simulink model "SCLAING_TRADITIONAL_21"  (R2021a)
settings: Solver=ode23tb  StartTime=0.0  StopTime=27  MaxStep=1/60  RelTol=1e-2  AbsTol=1e-1  EnableMultiTasking=on
PreLoadFcn:
  | NE39bus_data;
  | PSSMODEL=1;
  | LPSS=0;
  | WAPSS=0;
  | WAPSS2=0;
undefined symbols (not defined in the file): AVR_Data, D1, Delta, line, mac_con, MB, Ns, p0, Pn, s
libraries: spsThreePhaseVIMeasurementLib x40, spsThreePhasePISectionLineLib x34, spsGenericPowerSystemStabilizerLib x20, spsThreePhaseTransformerTwoWindingsLib x12, spsSynchronousMachinepuStandardLib x10, spsExcitationSystemLib x10, spsMultiBandPowerSystemStabilizerLib x10, spsSteamTurbineandGovernorLib x10, slpidlib x10, spsLoadFlowBusLib x9, spsThreePhaseDynamicLoadLib x9, spsThreePhaseParallelRLCLoadLib x9
(part 3 of 4)

== system SCLAING_TRADITIONAL_21/G8 ==
  DFG8 : Inport
  Bus Selector : BusSelector  OutputSignals="Mechanical.Rotor speed deviation  dw (pu)"
  Fcn2 : Fcn  Expr=60*(1+u)
  G8 : spsSynchronousMachinepuStandardLib/Synchronous Machine pu Standard  PresetModel=No  MechanicalLoad=Mechanical power Pm  ShowDetailedParameters=on  RotorType=Round  Units=per unit standard parameters  MeasurementBus=off  NominalParameters="[Pn(8,1)*1e9  22000   50 ]"  Reactances1="[mac_con(8,6:8)  mac_con(8,11:13)  mac_con(8,4)]"  Reactances2=[ 1.305, 0.296, 0.252, 0.474, 0.243, 0.18 ]  dAxisTimeConstants=Open-circuit  qAxisTimeConstants=Open-circuit  TimeConstants1=[]  TimeConstants2="[mac_con(8,9:10)  mac_con(8,14:15)]"  TimeConstants3=[]  TimeConstants4=[]  TimeConstants5=[ 1.01, 0.053, 0.1 ]  TimeConstants6=[]  TimeConstants7=[]  TimeConstants8=[]  StatorResistance=mac_con(8,5)  Mechanical="[ mac_con(8,16)  0  4]"  PolePairs=4  InitialConditions=[0 -25.6939 0.5409 0.5409 0.5409 6.7214 -113.279 126.721 1.90805]  SetSaturation=off  Saturation=[0.6404,0.7127,0.8441,0.9214,0.9956,1.082,1.19,1.316,1.457;0.7,0.7698,0.8872,0.9466,0.9969,1.046,1.1,1.151,1.201]  LoadFlowParameters=[1 540000000 0 0 0]  TsPowergui=0  TsBlock=-1  IterativeModel=Forward Euler  IterativeDiscreteModel=Trapezoidal non iterative  BusType=PV  Pref=p0(8,1)*1E9  Qref=0  Qmin=-inf  Qmax=inf  PLF=0  QLF=0
      settings: SourceProductBaseCode=PS
  M8: Turbine & Regulators : Subsystem
  Matrix Multiply1 : Product  Multiplication=Matrix(*)
  Matrix Multiply2 : Product  Multiplication=Matrix(*)
  PID Controller : slpidlib/PID Controller  Controller=PID  Form=Parallel  TimeDomain=Continuous-time  UseExternalTs=off  SampleTime=-1  IntegratorMethod=Forward Euler  FilterMethod=Forward Euler  ControllerParametersSource=internal  P=-0.20298  I=1  D=0  UseFilter=on  N=100  TunerSelectOption=Frequency Response Based  InitialConditionSource=internal  InitialConditionForIntegrator=0  InitialConditionForFilter=0  DifferentiatorICPrevScaledInput=0  ExternalReset=none  TrackingMode=off  Kt=1  LimitOutput=off  SatLimitsSource=internal  UpperSaturationLimit=inf  LowerSaturationLimit=-inf  LinearizeAsGain=on  AntiWindupMode=none  Kb=1  POutMin=[]  POutMax=[]  IOutMin=[]  IOutMax=[]  DOutMin=[]  DOutMax=[]  NOutMin=[]  NOutMax=[]  SumOutMin=[]  SumOutMax=[]  SaturationOutMin=[]  SaturationOutMax=[]  PParamMin=[]  PParamMax=[]  IParamMin=[]  IParamMax=[]  DParamMin=[]  DParamMax=[]  NParamMin=[]  NParamMax=[]  KbParamMin=[]  KbParamMax=[]  KtParamMin=[]  KtParamMax=[]  KbOutMin=[]  KbOutMax=[]  KtOutMin=[]  KtOutMax=[]  IntegratorOutMin=[]  IntegratorOutMax=[]  FilterOutMin=[]  FilterOutMax=[]  SumI1OutMin=[]  SumI1OutMax=[]  SumI2OutMin=[]  SumI2OutMax=[]  SumI3OutMin=[]  SumI3OutMax=[]  SumI4OutMin=[]  SumI4OutMax=[]  SumDOutMin=[]  SumDOutMax=[]  DifferentiatorOutMin=[]  DifferentiatorOutMax=[]  FilterDiffOutCoefMin=[]  FilterDiffOutCoefMax=[]  ReciprocalOutMin=[]  ReciprocalOutMax=[]  SumDenOutMin=[]  SumDenOutMax=[]  SumNumOutMin=[]  SumNumOutMax=[]  DivideOutMin=[]  DivideOutMax=[]  UdiffTsProdOutMin=[]  UdiffTsProdOutMax=[]  NTsProdOutMin=[]  NTsProdOutMax=[]  UintegralTsProdOutMin=[]  UintegralTsProdOutMax=[]  UngainTsProdOutMin=[]  UngainTsProdOutMax=[]  IntegratorContinuousStateAttributes=''  IntegratorStateMustResolveToSignalObject=off  IntegratorRTWStateStorageClass=Auto  FilterContinuousStateAttributes=''  FilterStateMustResolveToSignalObject=off  FilterRTWStateStorageClass=Auto  ParallelPVariant=InternalParameters  IdealPVariant=Disabled  IVariant=InternalParameters  DVariant=InternalParameters  IntegratorVariant=Continuous  SatVariant=Disabled  AWVariant=Passthrough  PCopyVariant=Disabled  TRVariant=Disabled  FdbkBlocksVariant=Forward  IdealPFdbkVariant=Disabled  SatFdbkVariant=Disabled  DerivativeFilterVariant=ContFilter  NVariant=InternalParameters  NCopyVariant=Disabled  FilterICVariant=InternalICsFilter  IntegratorICVariant=InternalICs  ExternalResetVariant=Disabled  TRSumVariant=Passthrough  SumFdbkVariant=Disabled  SumVariant=Sum_PID  TsampFilterVariant=InternalTs  TsampNgainVariant=Passthrough  TsampIntegralVariant=Passthrough  ExternalSaturationOutDataTypeStr=Inherit: Same as second input
  Pref8 : Constant  Value=0.54
  Scope : Scope
  Sum : Sum  Inputs=|++
  Vref8 : Constant
  A : PMIOPort  Side=Left
  B : PMIOPort  Port=2  Side=Left
  C : PMIOPort  Port=3  Side=Left
  GEN8 : Outport
  wires:
  G8/1 -> M8: Turbine & Regulators/1(m8), Bus Selector/1
  Vref8/1 -> M8: Turbine & Regulators/3(Vref8)
  [PSSmodel] -> M8: Turbine & Regulators/4(PSS8)
  Bus Selector/1 -> PID Controller/1, Fcn2/1  "<Rotor speed deviation  dw (pu)>"
  Fcn2/1 -> GEN8/1, Scope/1
  Pref8/1 -> Sum/1
  Sum/1 -> M8: Turbine & Regulators/2(Pref8)
  PID Controller/1 -> Sum/2
  DFG8/1 -> Matrix Multiply1/1, Matrix Multiply2/1
  M8: Turbine & Regulators/2(Vf8) -> Matrix Multiply2/2
  Matrix Multiply2/1 -> G8/2
  M8: Turbine & Regulators/1(Pm8) -> Matrix Multiply1/2
  Matrix Multiply1/1 -> G8/1
  connections:
  A/RConn1 -- G8/RConn1
  B/RConn1 -- G8/RConn2
  C/RConn1 -- G8/RConn3

== system SCLAING_TRADITIONAL_21/G9 ==
  DFG9 : Inport
  Bus Selector : BusSelector  OutputSignals="Mechanical.Rotor speed deviation  dw (pu)"
  Fcn2 : Fcn  Expr=60*(1+u)
  G9 : spsSynchronousMachinepuStandardLib/Synchronous Machine pu Standard  PresetModel=No  MechanicalLoad=Mechanical power Pm  ShowDetailedParameters=on  RotorType=Round  Units=per unit standard parameters  MeasurementBus=off  NominalParameters="[Pn(9,1)*1E9  22000   50 ]"  Reactances1="[mac_con(9,6:8)  mac_con(9,11:13)  mac_con(9,4)]"  Reactances2=[ 1.305, 0.296, 0.252, 0.474, 0.243, 0.18 ]  dAxisTimeConstants=Open-circuit  qAxisTimeConstants=Open-circuit  TimeConstants1=[]  TimeConstants2="[mac_con(9,9:10)  mac_con(9,14:15)]"  TimeConstants3=[]  TimeConstants4=[]  TimeConstants5=[ 1.01, 0.053, 0.1 ]  TimeConstants6=[]  TimeConstants7=[]  TimeConstants8=[]  StatorResistance=mac_con(9,5)  Mechanical="[ mac_con(9,16)  0  4]"  PolePairs=4  InitialConditions=[0 -16.7125 0.832308 0.832308 0.832308 12.5378 -107.462 132.538 2.08155]  SetSaturation=off  Saturation=[0.6404,0.7127,0.8441,0.9214,0.9956,1.082,1.19,1.316,1.457;0.7,0.7698,0.8872,0.9466,0.9969,1.046,1.1,1.151,1.201]  LoadFlowParameters=[1 830000000 0 0 0]  TsPowergui=0  TsBlock=-1  IterativeModel=Forward Euler  IterativeDiscreteModel=Trapezoidal non iterative  BusType=PV  Pref=p0(9,1)*1E9  Qref=0  Qmin=-inf  Qmax=inf  PLF=0  QLF=0
      settings: SourceProductBaseCode=PS
  "M9: Turbine & Regulators " : Subsystem
  Matrix Multiply1 : Product  Multiplication=Matrix(*)
  Matrix Multiply2 : Product  Multiplication=Matrix(*)
  PID Controller : slpidlib/PID Controller  Controller=PID  Form=Parallel  TimeDomain=Continuous-time  UseExternalTs=off  SampleTime=-1  IntegratorMethod=Forward Euler  FilterMethod=Forward Euler  ControllerParametersSource=internal  P=-0.20298  I=1  D=0  UseFilter=on  N=100  TunerSelectOption=Frequency Response Based  InitialConditionSource=internal  InitialConditionForIntegrator=0  InitialConditionForFilter=0  DifferentiatorICPrevScaledInput=0  ExternalReset=none  TrackingMode=off  Kt=1  LimitOutput=off  SatLimitsSource=internal  UpperSaturationLimit=inf  LowerSaturationLimit=-inf  LinearizeAsGain=on  AntiWindupMode=none  Kb=1  POutMin=[]  POutMax=[]  IOutMin=[]  IOutMax=[]  DOutMin=[]  DOutMax=[]  NOutMin=[]  NOutMax=[]  SumOutMin=[]  SumOutMax=[]  SaturationOutMin=[]  SaturationOutMax=[]  PParamMin=[]  PParamMax=[]  IParamMin=[]  IParamMax=[]  DParamMin=[]  DParamMax=[]  NParamMin=[]  NParamMax=[]  KbParamMin=[]  KbParamMax=[]  KtParamMin=[]  KtParamMax=[]  KbOutMin=[]  KbOutMax=[]  KtOutMin=[]  KtOutMax=[]  IntegratorOutMin=[]  IntegratorOutMax=[]  FilterOutMin=[]  FilterOutMax=[]  SumI1OutMin=[]  SumI1OutMax=[]  SumI2OutMin=[]  SumI2OutMax=[]  SumI3OutMin=[]  SumI3OutMax=[]  SumI4OutMin=[]  SumI4OutMax=[]  SumDOutMin=[]  SumDOutMax=[]  DifferentiatorOutMin=[]  DifferentiatorOutMax=[]  FilterDiffOutCoefMin=[]  FilterDiffOutCoefMax=[]  ReciprocalOutMin=[]  ReciprocalOutMax=[]  SumDenOutMin=[]  SumDenOutMax=[]  SumNumOutMin=[]  SumNumOutMax=[]  DivideOutMin=[]  DivideOutMax=[]  UdiffTsProdOutMin=[]  UdiffTsProdOutMax=[]  NTsProdOutMin=[]  NTsProdOutMax=[]  UintegralTsProdOutMin=[]  UintegralTsProdOutMax=[]  UngainTsProdOutMin=[]  UngainTsProdOutMax=[]  IntegratorContinuousStateAttributes=''  IntegratorStateMustResolveToSignalObject=off  IntegratorRTWStateStorageClass=Auto  FilterContinuousStateAttributes=''  FilterStateMustResolveToSignalObject=off  FilterRTWStateStorageClass=Auto  ParallelPVariant=InternalParameters  IdealPVariant=Disabled  IVariant=InternalParameters  DVariant=InternalParameters  IntegratorVariant=Continuous  SatVariant=Disabled  AWVariant=Passthrough  PCopyVariant=Disabled  TRVariant=Disabled  FdbkBlocksVariant=Forward  IdealPFdbkVariant=Disabled  SatFdbkVariant=Disabled  DerivativeFilterVariant=ContFilter  NVariant=InternalParameters  NCopyVariant=Disabled  FilterICVariant=InternalICsFilter  IntegratorICVariant=InternalICs  ExternalResetVariant=Disabled  TRSumVariant=Passthrough  SumFdbkVariant=Disabled  SumVariant=Sum_PID  TsampFilterVariant=InternalTs  TsampNgainVariant=Passthrough  TsampIntegralVariant=Passthrough  ExternalSaturationOutDataTypeStr=Inherit: Same as second input
  Pref9 : Constant  Value=0.83
  Scope : Scope
  Sum : Sum  Inputs=|++
  Vref9 : Constant
  A : PMIOPort  Side=Left
  B : PMIOPort  Port=2  Side=Left
  C : PMIOPort  Port=3  Side=Left
  Out1 : Outport
  GEN9 : Outport  Port=2
  wires:
  G9/1 -> Bus Selector/1, "M9: Turbine & Regulators "/1(m9)
  [PSSmodel] -> "M9: Turbine & Regulators "/4(PSS9)
  Vref9/1 -> "M9: Turbine & Regulators "/3(Vref9)
  Bus Selector/1 -> PID Controller/1, Fcn2/1  "<Rotor speed deviation  dw (pu)>"
  Fcn2/1 -> GEN9/1, Out1/1, Scope/1
  Pref9/1 -> Sum/1
  Sum/1 -> "M9: Turbine & Regulators "/2(Pref9)
  PID Controller/1 -> Sum/2
  DFG9/1 -> Matrix Multiply2/1, Matrix Multiply1/1
  "M9: Turbine & Regulators "/1(Pm9) -> Matrix Multiply1/2
  Matrix Multiply1/1 -> G9/1
  "M9: Turbine & Regulators "/2(Vf9) -> Matrix Multiply2/2
  Matrix Multiply2/1 -> G9/2
  connections:
  A/RConn1 -- G9/RConn1
  B/RConn1 -- G9/RConn2
  C/RConn1 -- G9/RConn3

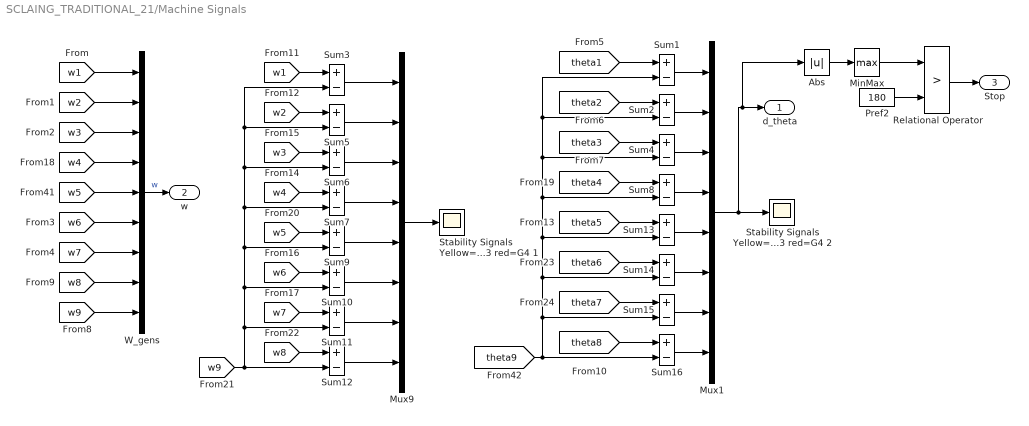
== system SCLAING_TRADITIONAL_21/Machine Signals ==
  Abs : Abs  SaturateOnIntegerOverflow=on
  MinMax : MinMax  Function=max  InputSameDT=on  SaturateOnIntegerOverflow=on
  Mux1 : Mux  Inputs=8
  Mux9 : Mux  Inputs=8
  Pref2 : Constant  Value=180
  Relational Operator : RelationalOperator  Operator=>  RndMeth=Nearest  InputSameDT=on
  Stability Signals Yellow=G1 mag=G2 cyan=G3 red=G4 1 : Scope
  Stability Signals Yellow=G1 mag=G2 cyan=G3 red=G4 2 : Scope
  Sum{1..16} (16 alike) : Sum  Inputs=+-  InputSameDT=on  SaturateOnIntegerOverflow=on  OutDataTypeStr=Inherit: Same as first input
  W_gens : Mux  Inputs=9
  d_theta : Outport
  w : Outport  Port=2
  Stop : Outport  Port=3
  wires:
  Abs/1 -> MinMax/1
  Pref2/1 -> Relational Operator/2
  MinMax/1 -> Relational Operator/1
  W_gens/1 -> w/1  "w"
  Relational Operator/1 -> Stop/1
  Mux9/1 -> Stability Signals Yellow=G1 mag=G2 cyan=G3 red=G4 1/1
  [w1] -> W_gens/1
  [w2] -> W_gens/2
  [w4] -> W_gens/4
  [w3] -> W_gens/3
  [w5] -> W_gens/5
  [w9] -> W_gens/9
  [w8] -> W_gens/8
  [w7] -> W_gens/7
  [w6] -> W_gens/6
  [w1] -> Sum3/1
  [w2] -> Sum5/1
  [w4] -> Sum7/1
  [w3] -> Sum6/1
  [w5] -> Sum9/1
  [w9] -> Sum11/2, Sum10/2, Sum9/2, Sum7/2, Sum6/2, Sum5/2, Sum3/2, Sum12/2
  [w8] -> Sum12/1
  [w7] -> Sum11/1
  [w6] -> Sum10/1
  Sum7/1 -> Mux9/4
  Sum6/1 -> Mux9/3
  Sum5/1 -> Mux9/2
  Sum3/1 -> Mux9/1
  Sum10/1 -> Mux9/6
  Sum9/1 -> Mux9/5
  Sum11/1 -> Mux9/7
  Sum12/1 -> Mux9/8
  [theta9] -> Sum15/2, Sum14/2, Sum4/2, Sum1/2, Sum2/2, Sum8/2, Sum13/2, Sum16/2
  [theta8] -> Sum16/1
  [theta1] -> Sum1/1
  [theta2] -> Sum2/1
  [theta3] -> Sum4/1
  [theta4] -> Sum8/1
  [theta5] -> Sum13/1
  [theta6] -> Sum14/1
  [theta7] -> Sum15/1
  Sum2/1 -> Mux1/2
  Sum1/1 -> Mux1/1
  Sum4/1 -> Mux1/3
  Sum8/1 -> Mux1/4
  Sum13/1 -> Mux1/5
  Sum14/1 -> Mux1/6
  Sum15/1 -> Mux1/7
  Sum16/1 -> Mux1/8
  Mux1/1 -> Abs/1, d_theta/1, Stability Signals Yellow=G1 mag=G2 cyan=G3 red=G4 2/1

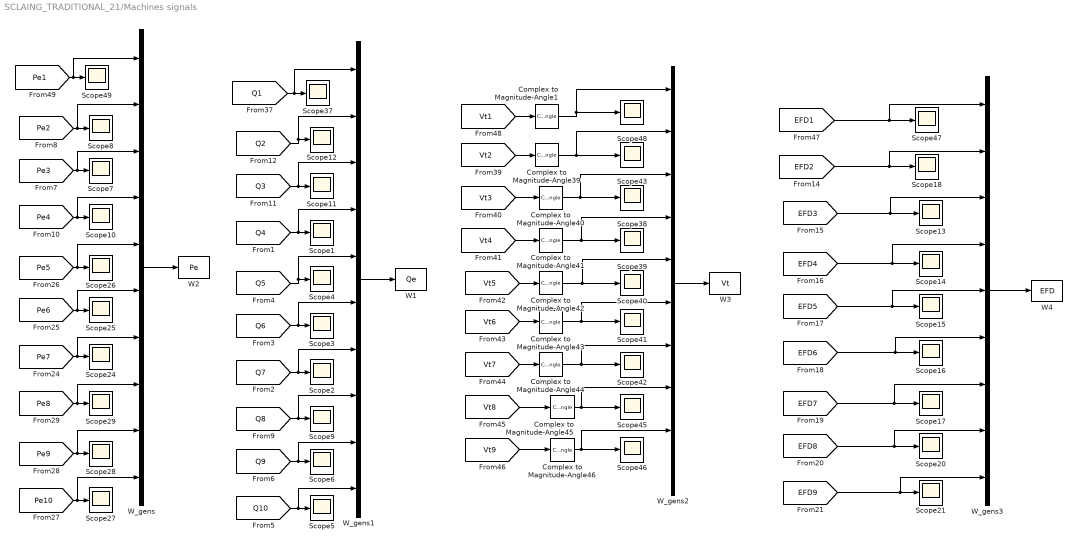
== system SCLAING_TRADITIONAL_21/Machines signals ==
  Complex to Magnitude-Angle{1,39..46} (9 alike) : ComplexToMagnitudeAngle  Output=Magnitude
  Scope{1..18,20..21,24..29,37..43,45..49} (38 alike) : Scope
  W1 : ToWorkspace  VariableName=Qe  SampleTime=1/60
  W2 : ToWorkspace  VariableName=Pe  SampleTime=1/60
  W3 : ToWorkspace  VariableName=Vt  SampleTime=1/60
  W4 : ToWorkspace  VariableName=EFD  SampleTime=1/60
  W_gens : Mux  Inputs=10
  W_gens1 : Mux  Inputs=10
  W_gens2 : Mux  Inputs=10
  W_gens3 : Mux  Inputs=9
  wires:
  [Pe3] -> W_gens/3, Scope7/1
  [Pe2] -> W_gens/2, Scope8/1
  [Vt2] -> Complex to Magnitude-Angle39/1
  Complex to Magnitude-Angle39/1 -> Scope43/1, W_gens2/2
  [Vt3] -> Complex to Magnitude-Angle40/1
  Complex to Magnitude-Angle40/1 -> Scope38/1, W_gens2/3
  [Vt4] -> Complex to Magnitude-Angle41/1
  Complex to Magnitude-Angle41/1 -> Scope39/1, W_gens2/4
  [Vt5] -> Complex to Magnitude-Angle42/1
  Complex to Magnitude-Angle42/1 -> Scope40/1, W_gens2/5
  [Vt6] -> Complex to Magnitude-Angle43/1
  Complex to Magnitude-Angle43/1 -> W_gens2/6, Scope41/1
  [Vt7] -> Complex to Magnitude-Angle44/1
  Complex to Magnitude-Angle44/1 -> Scope42/1, W_gens2/7
  [Vt8] -> Complex to Magnitude-Angle45/1
  Complex to Magnitude-Angle45/1 -> Scope45/1, W_gens2/8
  [Vt9] -> Complex to Magnitude-Angle46/1
  Complex to Magnitude-Angle46/1 -> W_gens2/9, Scope46/1
  [Pe6] -> W_gens/6, Scope25/1
  [Pe5] -> W_gens/5, Scope26/1
  [Pe7] -> W_gens/7, Scope24/1
  [Pe9] -> W_gens/9, Scope28/1
  [Pe8] -> W_gens/8, Scope29/1
  [Pe10] -> W_gens/10, Scope27/1
  [Q3] -> W_gens1/3, Scope11/1
  [Q2] -> W_gens1/2, Scope12/1
  [Q4] -> W_gens1/4, Scope1/1
  [Q6] -> W_gens1/6, Scope3/1
  [Q5] -> W_gens1/5, Scope4/1
  [Q7] -> W_gens1/7, Scope2/1
  [Q9] -> W_gens1/9, Scope6/1
  [Q8] -> W_gens1/8, Scope9/1
  [Q10] -> W_gens1/10, Scope5/1
  [EFD2] -> W_gens3/2, Scope18/1
  [EFD3] -> Scope13/1, W_gens3/3
  [EFD4] -> W_gens3/4, Scope14/1
  [EFD5] -> W_gens3/5, Scope15/1
  [EFD6] -> W_gens3/6, Scope16/1
  [EFD7] -> W_gens3/7, Scope17/1
  [EFD8] -> W_gens3/8, Scope20/1
  [EFD9] -> Scope21/1, W_gens3/9
  [Pe4] -> W_gens/4, Scope10/1
  [Pe1] -> W_gens/1, Scope49/1
  Complex to Magnitude-Angle1/1 -> W_gens2/1, Scope48/1
  [Q1] -> W_gens1/1, Scope37/1
  [EFD1] -> W_gens3/1, Scope47/1
  [Vt1] -> Complex to Magnitude-Angle1/1
  W_gens/1 -> W2/1
  W_gens1/1 -> W1/1
  W_gens2/1 -> W3/1
  W_gens3/1 -> W4/1

== system SCLAING_TRADITIONAL_21/Subsystem1 ==
  In3 : Inport
  Constant16 : Constant  Value=11304000  SampleTime=-1
  Constant17 : Constant  Value=0
  Matrix Multiply5 : Product  Multiplication=Matrix(*)
  Mux1 : Mux  Inputs=2
  Scope34 : Scope
  Sum4 : Sum  Inputs=|++
  Three-Phase Dynamic Load1 : spsThreePhaseDynamicLoadLib/Three-Phase Dynamic Load  NominalVoltage="[ (217684)*1  60 ]"  ActiveReactivePowers=[11304000 0]  PositiveSequence=[0.994 -11.8]  ExternalControl=on  NpNq=[1.3 2]  TimeConstants="[0  0  0  0]"  MinimumVoltage=0.7  Tfilter=-1  LoadFlowParameters=[4,0,0,0,0]
      settings: SourceProductBaseCode=PS
  Uniform Random Number1 : UniformRandomNumber  Minimum=-5e+3  Maximum=5e+3  Seed=1e+4  SampleTime=0.01
  A : PMIOPort  Side=Left
  B : PMIOPort  Port=2  Side=Left
  C : PMIOPort  Port=3  Side=Left
  m : Outport
  wires:
  Constant17/1 -> Mux1/2
  In3/1 -> Matrix Multiply5/1
  Matrix Multiply5/1 -> Scope34/1, Sum4/1
  Uniform Random Number1/1 -> Matrix Multiply5/2
  Three-Phase Dynamic Load1/1 -> m/1
  Sum4/1 -> Mux1/1
  Constant16/1 -> Sum4/2
  Mux1/1 -> Three-Phase Dynamic Load1/1
  connections:
  Three-Phase Dynamic Load1/LConn1 -- A/RConn1
  Three-Phase Dynamic Load1/LConn2 -- B/RConn1
  Three-Phase Dynamic Load1/LConn3 -- C/RConn1

== system SCLAING_TRADITIONAL_21/Subsystem2 ==
  In3 : Inport
  Constant16 : Constant  Value=11304000  SampleTime=-1
  Constant17 : Constant  Value=0
  Matrix Multiply5 : Product  Multiplication=Matrix(*)
  Mux1 : Mux  Inputs=2
  Scope34 : Scope
  Sum4 : Sum  Inputs=|++
  Three-Phase Dynamic Load1 : spsThreePhaseDynamicLoadLib/Three-Phase Dynamic Load  NominalVoltage="[ (217684)*1  60 ]"  ActiveReactivePowers=[11304000 0]  PositiveSequence=[0.994 -11.8]  ExternalControl=on  NpNq=[1.3 2]  TimeConstants="[0  0  0  0]"  MinimumVoltage=0.7  Tfilter=-1  LoadFlowParameters=[4,0,0,0,0]
      settings: SourceProductBaseCode=PS
  Uniform Random Number1 : UniformRandomNumber  Minimum=-5e+3  Maximum=5e+3  Seed=1e+4  SampleTime=0.01
  A : PMIOPort  Side=Left
  B : PMIOPort  Port=2  Side=Left
  C : PMIOPort  Port=3  Side=Left
  m : Outport
  wires:
  Constant17/1 -> Mux1/2
  In3/1 -> Matrix Multiply5/1
  Matrix Multiply5/1 -> Scope34/1, Sum4/1
  Uniform Random Number1/1 -> Matrix Multiply5/2
  Three-Phase Dynamic Load1/1 -> m/1
  Sum4/1 -> Mux1/1
  Constant16/1 -> Sum4/2
  Mux1/1 -> Three-Phase Dynamic Load1/1
  connections:
  Three-Phase Dynamic Load1/LConn1 -- A/RConn1
  Three-Phase Dynamic Load1/LConn2 -- B/RConn1
  Three-Phase Dynamic Load1/LConn3 -- C/RConn1

== system SCLAING_TRADITIONAL_21/Subsystem3 ==
  In3 : Inport
  Constant16 : Constant  Value=11304000  SampleTime=-1
  Constant17 : Constant  Value=0
  Matrix Multiply5 : Product  Multiplication=Matrix(*)
  Mux1 : Mux  Inputs=2
  Scope34 : Scope
  Sum4 : Sum  Inputs=|++
  Three-Phase Dynamic Load1 : spsThreePhaseDynamicLoadLib/Three-Phase Dynamic Load  NominalVoltage="[ (217684)*1  60 ]"  ActiveReactivePowers=[11304000 0]  PositiveSequence=[0.994 -11.8]  ExternalControl=on  NpNq=[1.3 2]  TimeConstants="[0  0  0  0]"  MinimumVoltage=0.7  Tfilter=-1  LoadFlowParameters=[4,0,0,0,0]
      settings: SourceProductBaseCode=PS
  Uniform Random Number1 : UniformRandomNumber  Minimum=-5e+3  Maximum=5e+3  Seed=1e+4  SampleTime=0.01
  A : PMIOPort  Side=Left
  B : PMIOPort  Port=2  Side=Left
  C : PMIOPort  Port=3  Side=Left
  m : Outport
  wires:
  Constant17/1 -> Mux1/2
  In3/1 -> Matrix Multiply5/1
  Matrix Multiply5/1 -> Scope34/1, Sum4/1
  Uniform Random Number1/1 -> Matrix Multiply5/2
  Three-Phase Dynamic Load1/1 -> m/1
  Sum4/1 -> Mux1/1
  Constant16/1 -> Sum4/2
  Mux1/1 -> Three-Phase Dynamic Load1/1
  connections:
  Three-Phase Dynamic Load1/LConn1 -- A/RConn1
  Three-Phase Dynamic Load1/LConn2 -- B/RConn1
  Three-Phase Dynamic Load1/LConn3 -- C/RConn1

== system SCLAING_TRADITIONAL_21/Subsystem4 ==
  In3 : Inport
  Constant16 : Constant  Value=11304000  SampleTime=-1
  Constant17 : Constant  Value=0
  Matrix Multiply5 : Product  Multiplication=Matrix(*)
  Mux1 : Mux  Inputs=2
  Scope34 : Scope
  Sum4 : Sum  Inputs=|++
  Three-Phase Dynamic Load1 : spsThreePhaseDynamicLoadLib/Three-Phase Dynamic Load  NominalVoltage="[ (217684)*1  60 ]"  ActiveReactivePowers=[11304000 0]  PositiveSequence=[0.994 -11.8]  ExternalControl=on  NpNq=[1.3 2]  TimeConstants="[0  0  0  0]"  MinimumVoltage=0.7  Tfilter=-1  LoadFlowParameters=[4,0,0,0,0]
      settings: SourceProductBaseCode=PS
  Uniform Random Number1 : UniformRandomNumber  Minimum=-5e+3  Maximum=5e+3  Seed=1e+4  SampleTime=0.01
  A : PMIOPort  Side=Left
  C : PMIOPort  Port=2  Side=Left
  B : PMIOPort  Port=3  Side=Left
  m : Outport
  wires:
  Constant17/1 -> Mux1/2
  In3/1 -> Matrix Multiply5/1
  Matrix Multiply5/1 -> Scope34/1, Sum4/1
  Uniform Random Number1/1 -> Matrix Multiply5/2
  Three-Phase Dynamic Load1/1 -> m/1
  Sum4/1 -> Mux1/1
  Constant16/1 -> Sum4/2
  Mux1/1 -> Three-Phase Dynamic Load1/1
  connections:
  Three-Phase Dynamic Load1/LConn1 -- A/RConn1
  Three-Phase Dynamic Load1/LConn2 -- B/RConn1
  Three-Phase Dynamic Load1/LConn3 -- C/RConn1

== system SCLAING_TRADITIONAL_21/Subsystem5 ==
  In3 : Inport
  Constant16 : Constant  Value=11304000  SampleTime=-1
  Constant17 : Constant  Value=0
  Matrix Multiply5 : Product  Multiplication=Matrix(*)
  Mux1 : Mux  Inputs=2
  Scope34 : Scope
  Sum4 : Sum  Inputs=|++
  Three-Phase Dynamic Load1 : spsThreePhaseDynamicLoadLib/Three-Phase Dynamic Load  NominalVoltage="[ (217684)*1  60 ]"  ActiveReactivePowers=[11304000 0]  PositiveSequence=[0.994 -11.8]  ExternalControl=on  NpNq=[1.3 2]  TimeConstants="[0  0  0  0]"  MinimumVoltage=0.7  Tfilter=-1  LoadFlowParameters=[4,0,0,0,0]
      settings: SourceProductBaseCode=PS
  Uniform Random Number1 : UniformRandomNumber  Minimum=-5e+3  Maximum=5e+3  Seed=1e+4  SampleTime=0.01
  A : PMIOPort  Side=Left
  B : PMIOPort  Port=2  Side=Left
  C : PMIOPort  Port=3  Side=Left
  m : Outport
  wires:
  Constant17/1 -> Mux1/2
  In3/1 -> Matrix Multiply5/1
  Matrix Multiply5/1 -> Scope34/1, Sum4/1
  Uniform Random Number1/1 -> Matrix Multiply5/2
  Three-Phase Dynamic Load1/1 -> m/1
  Sum4/1 -> Mux1/1
  Constant16/1 -> Sum4/2
  Mux1/1 -> Three-Phase Dynamic Load1/1
  connections:
  Three-Phase Dynamic Load1/LConn1 -- A/RConn1
  Three-Phase Dynamic Load1/LConn2 -- B/RConn1
  Three-Phase Dynamic Load1/LConn3 -- C/RConn1

== system SCLAING_TRADITIONAL_21/Subsystem6 ==
  In3 : Inport
  Constant16 : Constant  Value=11304000  SampleTime=-1
  Constant17 : Constant  Value=0
  Matrix Multiply5 : Product  Multiplication=Matrix(*)
  Mux1 : Mux  Inputs=2
  Scope34 : Scope
  Sum4 : Sum  Inputs=|++
  Three-Phase Dynamic Load1 : spsThreePhaseDynamicLoadLib/Three-Phase Dynamic Load  NominalVoltage="[ (217684)*1  60 ]"  ActiveReactivePowers=[11304000 0]  PositiveSequence=[0.994 -11.8]  ExternalControl=on  NpNq=[1.3 2]  TimeConstants="[0  0  0  0]"  MinimumVoltage=0.7  Tfilter=-1  LoadFlowParameters=[4,0,0,0,0]
      settings: SourceProductBaseCode=PS
  Uniform Random Number1 : UniformRandomNumber  Minimum=-5e+3  Maximum=5e+3  Seed=1e+4  SampleTime=0.01
  A : PMIOPort  Side=Left
  C : PMIOPort  Port=2  Side=Left
  B : PMIOPort  Port=3  Side=Left
  m : Outport
  wires:
  Constant17/1 -> Mux1/2
  In3/1 -> Matrix Multiply5/1
  Matrix Multiply5/1 -> Scope34/1, Sum4/1
  Uniform Random Number1/1 -> Matrix Multiply5/2
  Three-Phase Dynamic Load1/1 -> m/1
  Sum4/1 -> Mux1/1
  Constant16/1 -> Sum4/2
  Mux1/1 -> Three-Phase Dynamic Load1/1
  connections:
  Three-Phase Dynamic Load1/LConn1 -- A/RConn1
  Three-Phase Dynamic Load1/LConn2 -- B/RConn1
  Three-Phase Dynamic Load1/LConn3 -- C/RConn1

== system SCLAING_TRADITIONAL_21/Subsystem7 ==
  In3 : Inport
  Constant16 : Constant  Value=11304000  SampleTime=-1
  Constant17 : Constant  Value=0
  Matrix Multiply5 : Product  Multiplication=Matrix(*)
  Mux1 : Mux  Inputs=2
  Scope34 : Scope
  Sum4 : Sum  Inputs=|++
  Three-Phase Dynamic Load1 : spsThreePhaseDynamicLoadLib/Three-Phase Dynamic Load  NominalVoltage="[ (217684)*1  60 ]"  ActiveReactivePowers=[11304000 0]  PositiveSequence=[0.994 -11.8]  ExternalControl=on  NpNq=[1.3 2]  TimeConstants="[0  0  0  0]"  MinimumVoltage=0.7  Tfilter=-1  LoadFlowParameters=[4,0,0,0,0]
      settings: SourceProductBaseCode=PS
  Uniform Random Number1 : UniformRandomNumber  Minimum=-5e+3  Maximum=5e+3  Seed=1e+4  SampleTime=0.01
  A : PMIOPort  Side=Left
  B : PMIOPort  Port=2  Side=Left
  C : PMIOPort  Port=3  Side=Left
  m : Outport
  wires:
  Constant17/1 -> Mux1/2
  In3/1 -> Matrix Multiply5/1
  Matrix Multiply5/1 -> Scope34/1, Sum4/1
  Uniform Random Number1/1 -> Matrix Multiply5/2
  Three-Phase Dynamic Load1/1 -> m/1
  Sum4/1 -> Mux1/1
  Constant16/1 -> Sum4/2
  Mux1/1 -> Three-Phase Dynamic Load1/1
  connections:
  Three-Phase Dynamic Load1/LConn1 -- A/RConn1
  Three-Phase Dynamic Load1/LConn2 -- B/RConn1
  Three-Phase Dynamic Load1/LConn3 -- C/RConn1

== system SCLAING_TRADITIONAL_21/Subsystem8 ==
  In3 : Inport
  Constant16 : Constant  Value=11304000  SampleTime=-1
  Constant17 : Constant  Value=0
  Matrix Multiply5 : Product  Multiplication=Matrix(*)
  Mux1 : Mux  Inputs=2
  Scope34 : Scope
  Sum4 : Sum  Inputs=|++
  Three-Phase Dynamic Load1 : spsThreePhaseDynamicLoadLib/Three-Phase Dynamic Load  NominalVoltage="[ (217684)*1  60 ]"  ActiveReactivePowers=[11304000 0]  PositiveSequence=[0.994 -11.8]  ExternalControl=on  NpNq=[1.3 2]  TimeConstants="[0  0  0  0]"  MinimumVoltage=0.7  Tfilter=-1  LoadFlowParameters=[4,0,0,0,0]
      settings: SourceProductBaseCode=PS
  Uniform Random Number1 : UniformRandomNumber  Minimum=-5e+3  Maximum=5e+3  Seed=1e+4  SampleTime=0.01
  A : PMIOPort  Side=Left
  B : PMIOPort  Port=2  Side=Left
  C : PMIOPort  Port=3  Side=Left
  m : Outport
  wires:
  Constant17/1 -> Mux1/2
  In3/1 -> Matrix Multiply5/1
  Matrix Multiply5/1 -> Scope34/1, Sum4/1
  Uniform Random Number1/1 -> Matrix Multiply5/2
  Three-Phase Dynamic Load1/1 -> m/1
  Sum4/1 -> Mux1/1
  Constant16/1 -> Sum4/2
  Mux1/1 -> Three-Phase Dynamic Load1/1
  connections:
  Three-Phase Dynamic Load1/LConn1 -- A/RConn1
  Three-Phase Dynamic Load1/LConn2 -- B/RConn1
  Three-Phase Dynamic Load1/LConn3 -- C/RConn1

== system SCLAING_TRADITIONAL_21/Subsystem9 ==
  In3 : Inport
  Constant16 : Constant  Value=11304000  SampleTime=-1
  Constant17 : Constant  Value=0
  Matrix Multiply5 : Product  Multiplication=Matrix(*)
  Mux1 : Mux  Inputs=2
  Scope34 : Scope
  Sum4 : Sum  Inputs=|++
  Three-Phase Dynamic Load1 : spsThreePhaseDynamicLoadLib/Three-Phase Dynamic Load  NominalVoltage="[ (217684)*1  60 ]"  ActiveReactivePowers=[11304000 0]  PositiveSequence=[0.994 -11.8]  ExternalControl=on  NpNq=[1.3 2]  TimeConstants="[0  0  0  0]"  MinimumVoltage=0.7  Tfilter=-1  LoadFlowParameters=[4,0,0,0,0]
      settings: SourceProductBaseCode=PS
  Uniform Random Number1 : UniformRandomNumber  Minimum=-5e+3  Maximum=5e+3  Seed=1e+4  SampleTime=0.01
  A : PMIOPort  Side=Left
  C : PMIOPort  Port=2  Side=Left
  B : PMIOPort  Port=3  Side=Left
  m : Outport
  wires:
  Constant17/1 -> Mux1/2
  In3/1 -> Matrix Multiply5/1
  Matrix Multiply5/1 -> Scope34/1, Sum4/1
  Uniform Random Number1/1 -> Matrix Multiply5/2
  Three-Phase Dynamic Load1/1 -> m/1
  Sum4/1 -> Mux1/1
  Constant16/1 -> Sum4/2
  Mux1/1 -> Three-Phase Dynamic Load1/1
  connections:
  Three-Phase Dynamic Load1/LConn1 -- A/RConn1
  Three-Phase Dynamic Load1/LConn2 -- B/RConn1
  Three-Phase Dynamic Load1/LConn3 -- C/RConn1

== system SCLAING_TRADITIONAL_21/System Data ==
  ->pu : Gain  Gain=1/(230e3/sqrt(3)*sqrt(2))  SaturateOnIntegerOverflow=on  OutDataTypeStr=Inherit: Same as input  ParamDataTypeStr=Inherit: Same as input
  3-Phase Active & Reactive Power (Phasor Type) : powerlib_extras/Phasor Library/3-Phase Active & Reactive Power (Phasor Type)
      settings: SourceProductBaseCode=PS
  Complex to Magnitude-Angle : ComplexToMagnitudeAngle  Output=Magnitude
  Complex to Magnitude-Angle1 : ComplexToMagnitudeAngle  Output=Magnitude
  Mux : Mux  Inputs=2
  P34 : Gain  Gain=1e-6  SaturateOnIntegerOverflow=on  OutDataTypeStr=Inherit: Same as input  ParamDataTypeStr=Inherit: Same as input
  Selector : Selector  InputPortWidth=2  IndexOptions=Index vector (dialog)  Indices=1  OutputSizes=1
  Sequence Analyzer (Phasor Type) : powerlib_extras/Phasor Library/Sequence Analyzer (Phasor Type)  seq=Positive
      settings: SourceProductBaseCode=PS
  Sequence Analyzer (Phasor Type)1 : powerlib_extras/Phasor Library/Sequence Analyzer (Phasor Type)  seq=Positive
      settings: SourceProductBaseCode=PS
  Terminator1 : Terminator
  Terminator2 : Terminator
  Vabc_B3 : Scope
  Vabc_B4 : Scope
  W2 : ToWorkspace  VariableName=P21  SampleTime=1/60
  Vps : Outport
  p34 : Outport  Port=2
  wires:
  [Vabc_B4] -> Sequence Analyzer (Phasor Type)/1, 3-Phase Active & Reactive Power (Phasor Type)/1, Complex to Magnitude-Angle/1
  [Vabc_B3] -> Sequence Analyzer (Phasor Type)1/1, Complex to Magnitude-Angle1/1
  Sequence Analyzer (Phasor Type)/2 -> Terminator1/1
  Sequence Analyzer (Phasor Type)1/2 -> Terminator2/1
  Sequence Analyzer (Phasor Type)1/1 -> Mux/2
  [Iabc_B4] -> 3-Phase Active & Reactive Power (Phasor Type)/2
  3-Phase Active & Reactive Power (Phasor Type)/1 -> Selector/1
  ->pu/1 -> Vps/1
  Sequence Analyzer (Phasor Type)/1 -> Mux/1
  Mux/1 -> ->pu/1
  P34/1 -> p34/1, W2/1
  Complex to Magnitude-Angle/1 -> Vabc_B4/1
  Complex to Magnitude-Angle1/1 -> Vabc_B3/1
  Selector/1 -> P34/1

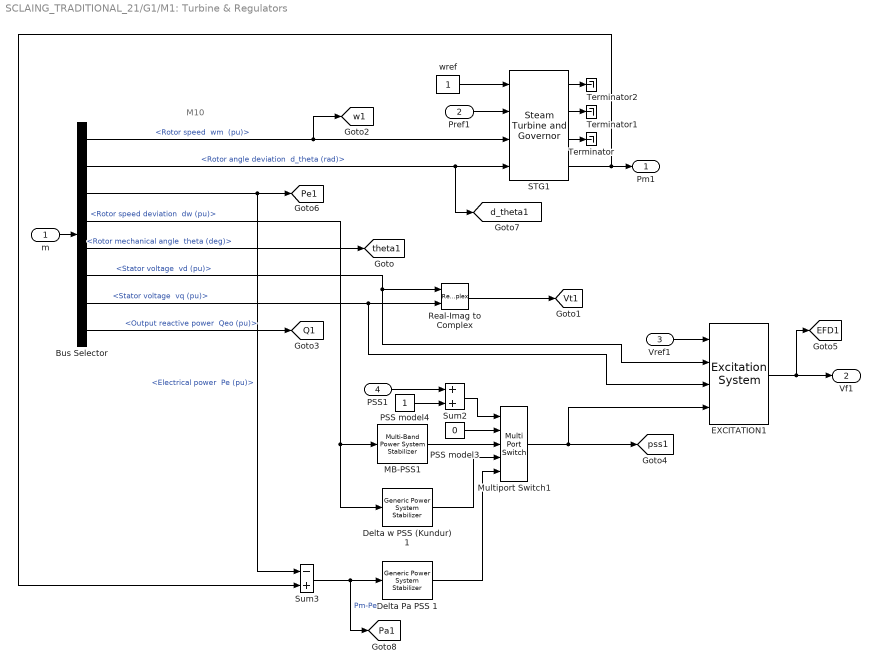
== system SCLAING_TRADITIONAL_21/G1/M1: Turbine & Regulators ==
  note: M10
  m : Inport
  Pref1 : Inport  Port=2
  Vref1 : Inport  Port=3
  PSS1 : Inport  Port=4
  Bus Selector : BusSelector  OutputSignals="Mechanical.Rotor speed  wm  (pu),Mechanical.Rotor angle deviation  d_theta (rad),Mechanical.Electrical power  Pe (pu),Mechanical.Rotor speed deviation  dw (pu),Mechanical.Rotor mechanical angle  theta (deg),dq0 components.Stator voltage  vd (pu),dq0 components.Stator voltage  vq (pu),Output reactive power  Qeo (pu)"
  Delta Pa PSS 1 : spsGenericPowerSystemStabilizerLib/Generic Power System Stabilizer  Tsensor=15e-3  K=2.5*1.25  Twashout=1  Tleadlag1=[60e-3 1]  Tleadlag2=[0 0]  VSlimits=[-0.15 0.15]  Vinit=0  Plot_On=off  MagdB_On=on  FreqRange=logspace(-2,2,500)
      settings: SourceProductBaseCode=PS
  Delta w PSS (Kundur) 1 : spsGenericPowerSystemStabilizerLib/Generic Power System Stabilizer  Tsensor=15e-3  K=30  Twashout=10  Tleadlag1=[50e-3 20e-3]  Tleadlag2=[3 5.4]  VSlimits=[-0.15 0.15]  Vinit=0  Plot_On=off  MagdB_On=on  FreqRange=logspace(-2,2,500)
      settings: SourceProductBaseCode=PS
  EXCITATION1 : spsExcitationSystemLib/Excitation System  tr=AVR_Data(1,1)  reg=[ AVR_Data(1,2:3) ]  exc=[ 1, 0 ]  tgr=[ AVR_Data(1,4:5)]  damp=[ 0, 0 ]  sat=[ 0, 0 ]  lim="[ AVR_Data(1,7:8)  0 ]"  v0=[1,1.07168]
      settings: SourceProductBaseCode=PS
  MB-PSS1 : spsMultiBandPowerSystemStabilizerLib/Multi-Band Power System Stabilizer  OperationMode=Simplified settings  Kg=MB(1)  GL=[MB(2) MB(3)]  GI=[MB(4) MB(5)]  GH=[MB(6) MB(7)]  GLd=[66 66 9.4]  TcLF=[1.667 2 0 0 0 0 2 2.4 0 0 0 0 1 1]  GId=[66 66 47.6]  TcIF=[1 1 0.25 0.3 0 0 1 1 0.3 0.36 0 0 0 0]  GHd=[66 66 233]  TcHF="[0.01 0.012 0 0 0 0  0.012 0.0144 0 0 0 0 1 1]"  LIM=[.075 .15 .15 .15]  Plot_On=off  MagdB_On=off  FreqRange=logspace(-2,2,500)
      settings: SourceProductBaseCode=PS
  Multiport Switch1 : MultiPortSwitch  Inputs=4  InputSameDT=on
  PSS model3 : Constant  Value=0
  PSS model4 : Constant
  Real-Imag to Complex : RealImagToComplex
  STG1 : spsSteamTurbineandGovernorLib/Steam Turbine and Governor  gentype=Tandem-compound (single mass)  reg1="[ 1  0.05    0 ]"  reg2="[ 0.001  0.15 ]"  reg3="[ -0.1  0.1  0  4.496 ]"  N=Ns  turb1="[ 0  10   3.3   0.5   ]"  turb2="[   0   0.36    0.36   0.28   ]"  HA="[ 0.046  1.430  1.465   0.192 ]"  KA="[ 90.44  53.88  64.59   62.94  ]"  DA="[ 0.0115  0.3575  0.3663   0.0137  ]"  ini1=1  ini2=[0.779316,-31.4247]
      settings: SourceProductBaseCode=PS
  Sum2 : Sum  InputSameDT=on  SaturateOnIntegerOverflow=on  OutDataTypeStr=Inherit: Same as first input
  Sum3 : Sum  Inputs=-+  InputSameDT=on  SaturateOnIntegerOverflow=on  OutDataTypeStr=Inherit: Same as first input
  Terminator : Terminator
  Terminator1 : Terminator
  Terminator2 : Terminator
  wref : Constant
  Pm1 : Outport  InitialOutput=0
  Vf1 : Outport  Port=2  InitialOutput=0
  tag scope: EFD1=global, Pa1=global, Pe1=global, Q1=global, Vt1=global, d_theta1=global, pss1=global, theta1=global, w1=global
  wires:
  Bus Selector/7 -> EXCITATION1/3, Real-Imag to Complex/2  "<Stator voltage  vq (pu)>"
  wref/1 -> STG1/1
  Pref1/1 -> STG1/2
  m/1 -> Bus Selector/1
  Vref1/1 -> EXCITATION1/1
  EXCITATION1/1 -> Vf1/1, [EFD1]
  Real-Imag to Complex/1 -> [Vt1]
  Bus Selector/5 -> [theta1]  "<Rotor mechanical angle  theta (deg)>"
  Bus Selector/6 -> Real-Imag to Complex/1, EXCITATION1/2  "<Stator voltage  vd (pu)>"
  STG1/3 -> Terminator/1
  STG1/4 -> Sum3/2, Pm1/1
  STG1/2 -> Terminator1/1
  STG1/1 -> Terminator2/1
  Bus Selector/1 -> [w1], STG1/3  "<Rotor speed  wm  (pu)>"
  Bus Selector/2 -> [d_theta1], STG1/4  "<Rotor angle deviation  d_theta (rad)>"
  Bus Selector/3 -> Sum3/1, [Pe1]  "<Electrical power  Pe (pu)>"
  Bus Selector/8 -> [Q1]  "<Output reactive power  Qeo (pu)>"
  Sum3/1 -> [Pa1], Delta Pa PSS 1/1  "Pm-Pe"
  PSS1/1 -> Sum2/1
  Sum2/1 -> Multiport Switch1/1
  PSS model4/1 -> Sum2/2
  Delta Pa PSS 1/1 -> Multiport Switch1/5
  Delta w PSS (Kundur) 1/1 -> Multiport Switch1/4
  MB-PSS1/1 -> Multiport Switch1/3
  PSS model3/1 -> Multiport Switch1/2
  Multiport Switch1/1 -> [pss1], EXCITATION1/4
  Bus Selector/4 -> Delta w PSS (Kundur) 1/1, MB-PSS1/1  "<Rotor speed deviation  dw (pu)>"

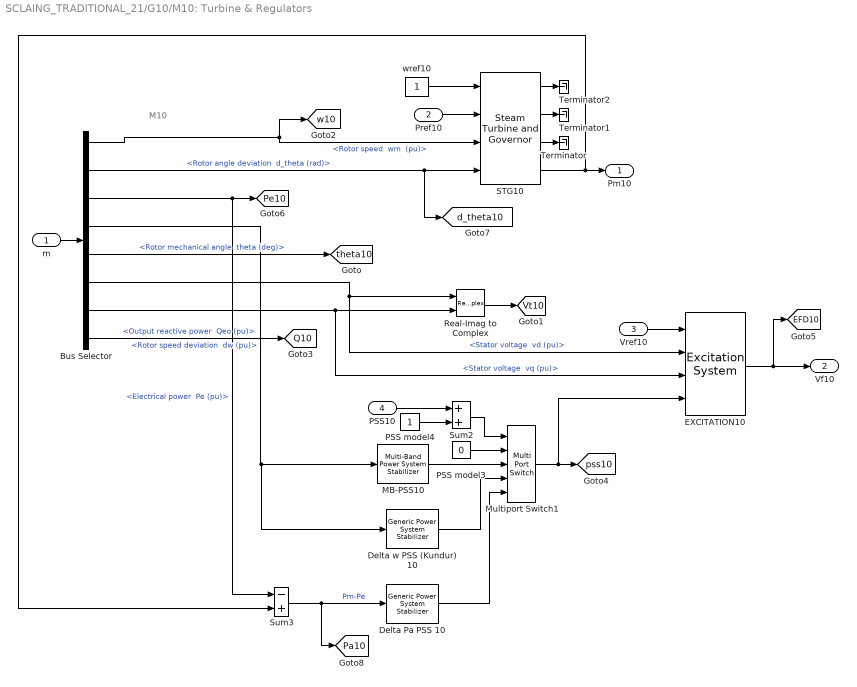
== system SCLAING_TRADITIONAL_21/G10/M10: Turbine & Regulators ==
  note: M10
  m : Inport
  Pref10 : Inport  Port=2
  Vref10 : Inport  Port=3
  PSS10 : Inport  Port=4
  Bus Selector : BusSelector  OutputSignals="Mechanical.Rotor speed  wm  (pu),Mechanical.Rotor angle deviation  d_theta (rad),Mechanical.Electrical power  Pe (pu),Mechanical.Rotor speed deviation  dw (pu),Mechanical.Rotor mechanical angle  theta (deg),dq0 components.Stator voltage  vd (pu),dq0 components.Stator voltage  vq (pu),Output reactive power  Qeo (pu)"
  Delta Pa PSS 10 : spsGenericPowerSystemStabilizerLib/Generic Power System Stabilizer  Tsensor=15e-3  K=2.5*1.25  Twashout=1  Tleadlag1=[60e-3 1]  Tleadlag2=[0 0]  VSlimits=[-0.15 0.15]  Vinit=0  Plot_On=off  MagdB_On=on  FreqRange=logspace(-2,2,500)
      settings: SourceProductBaseCode=PS
  Delta w PSS (Kundur) 10 : spsGenericPowerSystemStabilizerLib/Generic Power System Stabilizer  Tsensor=15e-3  K=30  Twashout=10  Tleadlag1=[50e-3 20e-3]  Tleadlag2=[3 5.4]  VSlimits=[-0.15 0.15]  Vinit=0  Plot_On=off  MagdB_On=on  FreqRange=logspace(-2,2,500)
      settings: SourceProductBaseCode=PS
  EXCITATION10 : spsExcitationSystemLib/Excitation System  tr=AVR_Data(1,1)  reg=[ AVR_Data(1,2:3) ]  exc=[ 1, 0 ]  tgr=[ AVR_Data(1,4:5)]  damp=[ 0, 0 ]  sat=[ 0, 0 ]  lim="[ AVR_Data(1,7:8)  0 ]"  v0=[1,1.1157]
      settings: SourceProductBaseCode=PS
  "MB-PSS10 " : spsMultiBandPowerSystemStabilizerLib/Multi-Band Power System Stabilizer  OperationMode=Simplified settings  Kg=MB(1)  GL=[MB(2) MB(3)]  GI=[MB(4) MB(5)]  GH=[MB(6) MB(7)]  GLd=[66 66 9.4]  TcLF=[1.667 2 0 0 0 0 2 2.4 0 0 0 0 1 1]  GId=[66 66 47.6]  TcIF=[1 1 0.25 0.3 0 0 1 1 0.3 0.36 0 0 0 0]  GHd=[66 66 233]  TcHF="[0.01 0.012 0 0 0 0  0.012 0.0144 0 0 0 0 1 1]"  LIM=[.075 .15 .15 .15]  Plot_On=off  MagdB_On=off  FreqRange=logspace(-2,2,500)
      settings: SourceProductBaseCode=PS
  Multiport Switch1 : MultiPortSwitch  Inputs=4  InputSameDT=on
  PSS model3 : Constant  Value=0
  PSS model4 : Constant
  Real-Imag to Complex : RealImagToComplex
  STG10 : spsSteamTurbineandGovernorLib/Steam Turbine and Governor  gentype=Tandem-compound (single mass)  reg1="[ 1  0.05    0 ]"  reg2="[ 0.001  0.15 ]"  reg3="[ -0.1  0.1  0  4.496 ]"  N=Ns  turb1="[ 0  10   3.3   0.5   ]"  turb2="[   0   0.36    0.36   0.28   ]"  HA="[ 0.046  1.430  1.465   0.192 ]"  KA="[ 90.44  53.88  64.59   62.94  ]"  DA="[ 0.0115  0.3575  0.3663   0.0137  ]"  ini1=0.25  ini2=[0.779316,-31.4247]
      settings: SourceProductBaseCode=PS
  Sum2 : Sum  InputSameDT=on  SaturateOnIntegerOverflow=on  OutDataTypeStr=Inherit: Same as first input
  Sum3 : Sum  Inputs=-+  InputSameDT=on  SaturateOnIntegerOverflow=on  OutDataTypeStr=Inherit: Same as first input
  Terminator : Terminator
  Terminator1 : Terminator
  Terminator2 : Terminator
  wref10 : Constant
  Pm10 : Outport  InitialOutput=0
  Vf10 : Outport  Port=2  InitialOutput=0
  tag scope: EFD10=global, Pa10=global, Pe10=global, Q10=global, Vt10=global, d_theta10=global, pss10=global, theta10=global, w10=global
  wires:
  Bus Selector/7 -> EXCITATION10/3, Real-Imag to Complex/2  "<Stator voltage  vq (pu)>"
  wref10/1 -> STG10/1
  Pref10/1 -> STG10/2
  m/1 -> Bus Selector/1
  Vref10/1 -> EXCITATION10/1
  EXCITATION10/1 -> Vf10/1, [EFD10]
  Real-Imag to Complex/1 -> [Vt10]
  Bus Selector/5 -> [theta10]  "<Rotor mechanical angle  theta (deg)>"
  Bus Selector/6 -> Real-Imag to Complex/1, EXCITATION10/2  "<Stator voltage  vd (pu)>"
  STG10/3 -> Terminator/1
  STG10/4 -> Sum3/2, Pm10/1
  STG10/2 -> Terminator1/1
  STG10/1 -> Terminator2/1
  Bus Selector/1 -> STG10/3, [w10]  "<Rotor speed  wm  (pu)>"
  Bus Selector/2 -> [d_theta10], STG10/4  "<Rotor angle deviation  d_theta (rad)>"
  Bus Selector/3 -> Sum3/1, [Pe10]  "<Electrical power  Pe (pu)>"
  Bus Selector/4 -> Delta w PSS (Kundur) 10/1, "MB-PSS10 "/1  "<Rotor speed deviation  dw (pu)>"
  Bus Selector/8 -> [Q10]  "<Output reactive power  Qeo (pu)>"
  Sum3/1 -> Delta Pa PSS 10/1, [Pa10]  "Pm-Pe"
  Sum2/1 -> Multiport Switch1/1
  PSS model4/1 -> Sum2/2
  Delta Pa PSS 10/1 -> Multiport Switch1/5
  Delta w PSS (Kundur) 10/1 -> Multiport Switch1/4
  "MB-PSS10 "/1 -> Multiport Switch1/3
  PSS model3/1 -> Multiport Switch1/2
  Multiport Switch1/1 -> EXCITATION10/4, [pss10]
  PSS10/1 -> Sum2/1

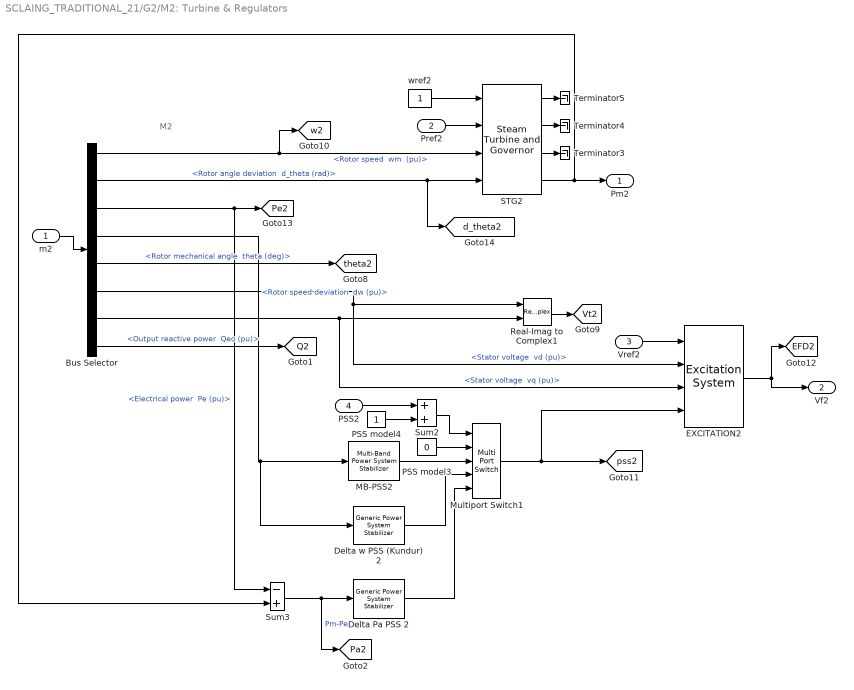
== system SCLAING_TRADITIONAL_21/G2/M2: Turbine & Regulators ==
  note: M2
  m2 : Inport
  Pref2 : Inport  Port=2
  Vref2 : Inport  Port=3
  PSS2 : Inport  Port=4
  Bus Selector : BusSelector  OutputSignals="Mechanical.Rotor speed  wm  (pu),Mechanical.Rotor angle deviation  d_theta (rad),Mechanical.Electrical power  Pe (pu),Mechanical.Rotor speed deviation  dw (pu),Mechanical.Rotor mechanical angle  theta (deg),dq0 components.Stator voltage  vd (pu),dq0 components.Stator voltage  vq (pu),Output reactive power  Qeo (pu)"
  Delta Pa PSS 2 : spsGenericPowerSystemStabilizerLib/Generic Power System Stabilizer  Tsensor=15e-3  K=2.5*1.25  Twashout=1  Tleadlag1=[60e-3 1]  Tleadlag2=[0 0]  VSlimits=[-0.15 0.15]  Vinit=0  Plot_On=off  MagdB_On=on  FreqRange=logspace(-2,2,500)
      settings: SourceProductBaseCode=PS
  Delta w PSS (Kundur) 2 : spsGenericPowerSystemStabilizerLib/Generic Power System Stabilizer  Tsensor=15e-3  K=30  Twashout=10  Tleadlag1=[50e-3 20e-3]  Tleadlag2=[3 5.4]  VSlimits=[-0.15 0.15]  Vinit=0  Plot_On=off  MagdB_On=on  FreqRange=logspace(-2,2,500)
      settings: SourceProductBaseCode=PS
  EXCITATION2 : spsExcitationSystemLib/Excitation System  tr=AVR_Data(2,1)  reg=[ AVR_Data(2,2:3) ]  exc=[ 1, 0 ]  tgr=[ AVR_Data(2,4:5)]  damp=[ 0, 0 ]  sat=[ 0, 0 ]  lim="[ AVR_Data(2,7:8)  0 ]"  v0=[1,1.77729]
      settings: SourceProductBaseCode=PS
  MB-PSS2 : spsMultiBandPowerSystemStabilizerLib/Multi-Band Power System Stabilizer  OperationMode=Simplified settings  Kg=MB(1)  GL=[MB(2) MB(3)]  GI=[MB(4) MB(5)]  GH=[MB(6) MB(7)]  GLd=[66 66 9.4]  TcLF=[1.667 2 0 0 0 0 2 2.4 0 0 0 0 1 1]  GId=[66 66 47.6]  TcIF=[1 1 0.25 0.3 0 0 1 1 0.3 0.36 0 0 0 0]  GHd=[66 66 233]  TcHF="[0.01 0.012 0 0 0 0  0.012 0.0144 0 0 0 0 1 1]"  LIM=[.075 .15 .15 .15]  Plot_On=off  MagdB_On=off  FreqRange=logspace(-2,2,500)
      settings: SourceProductBaseCode=PS
  Multiport Switch1 : MultiPortSwitch  Inputs=4  InputSameDT=on
  PSS model3 : Constant  Value=0
  PSS model4 : Constant
  Real-Imag to Complex1 : RealImagToComplex
  STG2 : spsSteamTurbineandGovernorLib/Steam Turbine and Governor  gentype=Tandem-compound (single mass)  reg1="[ 1  0.05    0 ]"  reg2="[ 0.001  0.15 ]"  reg3="[ -0.1  0.1  0  4.496 ]"  N=Ns  turb1="[ 0  10   3.3   0.5   ]"  turb2="[   0   0.36    0.36   0.28   ]"  HA="[ 0.046  1.430  1.465   0.192 ]"  KA="[ 90.44  53.88  64.59   62.94  ]"  DA="[ 0.0115  0.3575  0.3663   0.0137  ]"  ini1=0.277303  ini2=[0.779316,-31.4247]
      settings: SourceProductBaseCode=PS
  Sum2 : Sum  InputSameDT=on  SaturateOnIntegerOverflow=on  OutDataTypeStr=Inherit: Same as first input
  Sum3 : Sum  Inputs=-+  InputSameDT=on  SaturateOnIntegerOverflow=on  OutDataTypeStr=Inherit: Same as first input
  Terminator3 : Terminator
  Terminator4 : Terminator
  Terminator5 : Terminator
  wref2 : Constant
  Pm2 : Outport  InitialOutput=0
  Vf2 : Outport  Port=2  InitialOutput=0
  tag scope: EFD2=global, Pa2=global, Pe2=global, Q2=global, Vt2=global, d_theta2=global, pss2=global, theta2=global, w2=global
  wires:
  Bus Selector/7 -> EXCITATION2/3, Real-Imag to Complex1/2  "<Stator voltage  vq (pu)>"
  wref2/1 -> STG2/1
  Pref2/1 -> STG2/2
  m2/1 -> Bus Selector/1
  Vref2/1 -> EXCITATION2/1
  EXCITATION2/1 -> Vf2/1, [EFD2]
  Real-Imag to Complex1/1 -> [Vt2]
  Bus Selector/5 -> [theta2]  "<Rotor mechanical angle  theta (deg)>"
  Bus Selector/6 -> EXCITATION2/2, Real-Imag to Complex1/1  "<Stator voltage  vd (pu)>"
  STG2/3 -> Terminator3/1
  STG2/4 -> Sum3/2, Pm2/1
  STG2/2 -> Terminator4/1
  STG2/1 -> Terminator5/1
  Bus Selector/1 -> [w2], STG2/3  "<Rotor speed  wm  (pu)>"
  Bus Selector/2 -> [d_theta2], STG2/4  "<Rotor angle deviation  d_theta (rad)>"
  Bus Selector/3 -> Sum3/1, [Pe2]  "<Electrical power  Pe (pu)>"
  Bus Selector/4 -> Delta w PSS (Kundur) 2/1, MB-PSS2/1  "<Rotor speed deviation  dw (pu)>"
  Bus Selector/8 -> [Q2]  "<Output reactive power  Qeo (pu)>"
  Sum3/1 -> [Pa2], Delta Pa PSS 2/1  "Pm-Pe"
  Sum2/1 -> Multiport Switch1/1
  PSS model4/1 -> Sum2/2
  Delta Pa PSS 2/1 -> Multiport Switch1/5
  Delta w PSS (Kundur) 2/1 -> Multiport Switch1/4
  MB-PSS2/1 -> Multiport Switch1/3
  PSS model3/1 -> Multiport Switch1/2
  Multiport Switch1/1 -> [pss2], EXCITATION2/4
  PSS2/1 -> Sum2/1

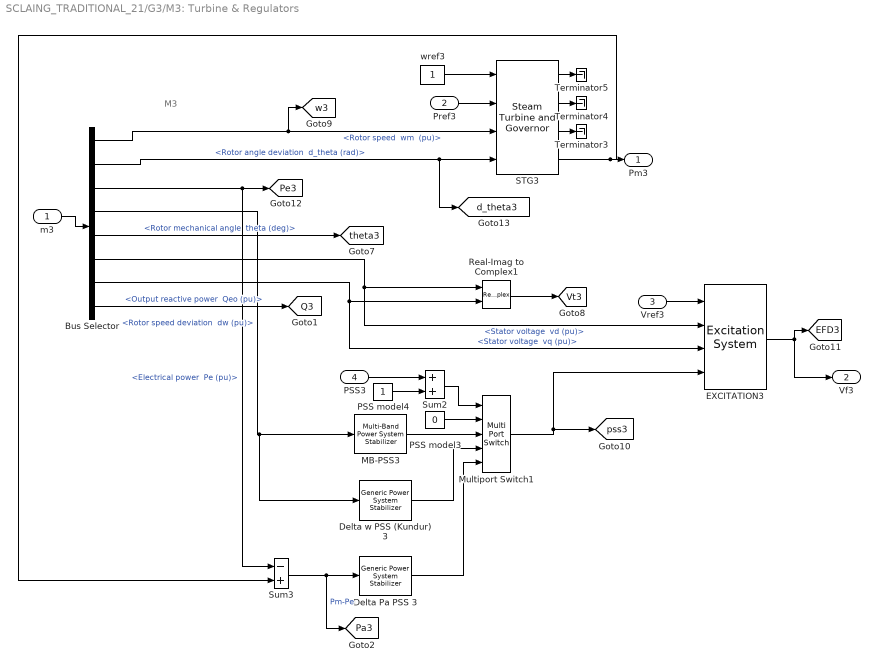
== system SCLAING_TRADITIONAL_21/G3/M3: Turbine & Regulators ==
  note: M3
  m3 : Inport
  Pref3 : Inport  Port=2
  Vref3 : Inport  Port=3
  PSS3 : Inport  Port=4
  Bus Selector : BusSelector  OutputSignals="Mechanical.Rotor speed  wm  (pu),Mechanical.Rotor angle deviation  d_theta (rad),Mechanical.Electrical power  Pe (pu),Mechanical.Rotor speed deviation  dw (pu),Mechanical.Rotor mechanical angle  theta (deg),dq0 components.Stator voltage  vd (pu),dq0 components.Stator voltage  vq (pu),Output reactive power  Qeo (pu)"
  Delta Pa PSS 3 : spsGenericPowerSystemStabilizerLib/Generic Power System Stabilizer  Tsensor=15e-3  K=2.5*1.25  Twashout=1  Tleadlag1=[60e-3 1]  Tleadlag2=[0 0]  VSlimits=[-0.15 0.15]  Vinit=0  Plot_On=off  MagdB_On=on  FreqRange=logspace(-2,2,500)
      settings: SourceProductBaseCode=PS
  Delta w PSS (Kundur) 3 : spsGenericPowerSystemStabilizerLib/Generic Power System Stabilizer  Tsensor=15e-3  K=30  Twashout=10  Tleadlag1=[50e-3 20e-3]  Tleadlag2=[3 5.4]  VSlimits=[-0.15 0.15]  Vinit=0  Plot_On=off  MagdB_On=on  FreqRange=logspace(-2,2,500)
      settings: SourceProductBaseCode=PS
  EXCITATION3 : spsExcitationSystemLib/Excitation System  tr=AVR_Data(3,1)  reg=[ AVR_Data(3,2:3) ]  exc=[ 1, 0 ]  tgr=[ AVR_Data(3,4:5)]  damp=[ 0, 0 ]  sat=[ 0, 0 ]  lim="[ AVR_Data(3,7:8)  0 ]"  v0=[1,2.25944]
      settings: SourceProductBaseCode=PS
  MB-PSS3 : spsMultiBandPowerSystemStabilizerLib/Multi-Band Power System Stabilizer  OperationMode=Simplified settings  Kg=MB(1)  GL=[MB(2) MB(3)]  GI=[MB(4) MB(5)]  GH=[MB(6) MB(7)]  GLd=[66 66 9.4]  TcLF=[1.667 2 0 0 0 0 2 2.4 0 0 0 0 1 1]  GId=[66 66 47.6]  TcIF=[1 1 0.25 0.3 0 0 1 1 0.3 0.36 0 0 0 0]  GHd=[66 66 233]  TcHF="[0.01 0.012 0 0 0 0  0.012 0.0144 0 0 0 0 1 1]"  LIM=[.075 .15 .15 .15]  Plot_On=off  MagdB_On=off  FreqRange=logspace(-2,2,500)
      settings: SourceProductBaseCode=PS
  Multiport Switch1 : MultiPortSwitch  Inputs=4  InputSameDT=on
  PSS model3 : Constant  Value=0
  PSS model4 : Constant
  Real-Imag to Complex1 : RealImagToComplex
  STG3 : spsSteamTurbineandGovernorLib/Steam Turbine and Governor  gentype=Tandem-compound (single mass)  reg1="[ 1  0.05    0 ]"  reg2="[ 0.001  0.15 ]"  reg3="[ -0.1  0.1  0  4.496 ]"  N=Ns  turb1="[ 0  10   3.3   0.5   ]"  turb2="[   0   0.36    0.36   0.28   ]"  HA="[ 0.046  1.430  1.465   0.192 ]"  KA="[ 90.44  53.88  64.59   62.94  ]"  DA="[ 0.0115  0.3575  0.3663   0.0137  ]"  ini1=0.65  ini2=[0.779316,-31.4247]
      settings: SourceProductBaseCode=PS
  Sum2 : Sum  InputSameDT=on  SaturateOnIntegerOverflow=on  OutDataTypeStr=Inherit: Same as first input
  Sum3 : Sum  Inputs=-+  InputSameDT=on  SaturateOnIntegerOverflow=on  OutDataTypeStr=Inherit: Same as first input
  Terminator3 : Terminator
  Terminator4 : Terminator
  Terminator5 : Terminator
  wref3 : Constant
  Pm3 : Outport  InitialOutput=0
  Vf3 : Outport  Port=2  InitialOutput=0
  tag scope: EFD3=global, Pa3=global, Pe3=global, Q3=global, Vt3=global, d_theta3=global, pss3=global, theta3=global, w3=global
  wires:
  Bus Selector/7 -> EXCITATION3/3, Real-Imag to Complex1/2  "<Stator voltage  vq (pu)>"
  wref3/1 -> STG3/1
  Pref3/1 -> STG3/2
  m3/1 -> Bus Selector/1
  Vref3/1 -> EXCITATION3/1
  EXCITATION3/1 -> Vf3/1, [EFD3]
  Real-Imag to Complex1/1 -> [Vt3]
  Bus Selector/5 -> [theta3]  "<Rotor mechanical angle  theta (deg)>"
  Bus Selector/6 -> EXCITATION3/2, Real-Imag to Complex1/1  "<Stator voltage  vd (pu)>"
  STG3/3 -> Terminator3/1
  STG3/4 -> Sum3/2, Pm3/1
  STG3/2 -> Terminator4/1
  STG3/1 -> Terminator5/1
  Bus Selector/1 -> [w3], STG3/3  "<Rotor speed  wm  (pu)>"
  Bus Selector/2 -> STG3/4, [d_theta3]  "<Rotor angle deviation  d_theta (rad)>"
  Bus Selector/3 -> Sum3/1, [Pe3]  "<Electrical power  Pe (pu)>"
  Bus Selector/4 -> Delta w PSS (Kundur) 3/1, MB-PSS3/1  "<Rotor speed deviation  dw (pu)>"
  Bus Selector/8 -> [Q3]  "<Output reactive power  Qeo (pu)>"
  Sum3/1 -> [Pa3], Delta Pa PSS 3/1  "Pm-Pe"
  Sum2/1 -> Multiport Switch1/1
  PSS model4/1 -> Sum2/2
  Delta Pa PSS 3/1 -> Multiport Switch1/5
  Delta w PSS (Kundur) 3/1 -> Multiport Switch1/4
  MB-PSS3/1 -> Multiport Switch1/3
  PSS model3/1 -> Multiport Switch1/2
  Multiport Switch1/1 -> EXCITATION3/4, [pss3]
  PSS3/1 -> Sum2/1
